simulink model "Controller_ABS_VLC_AYC"  (Simulink 8.7)
settings: Solver=ode3  SolverMode=SingleTasking  StartTime=0.0  StopTime=6  FixedStep=0.001  RelTol=1e-3
undefined symbols (not defined in the file): Lf, Lr, T_Avail
libraries: fuzblock x17, slrtlib x10, dspfdesign x5, simulink x4
settings Model: MinMaxOverflowLogging=ForceOff  Creator=MR Spyder  LastModifiedBy=kschmutz
settings DataIOCC: SignalLoggingSaveFormat=ModelDataLogs  SaveOutput=off  SaveTime=off
settings OptimizationCC: DefaultParameterBehavior=Inlined  ExpressionDepthLimit=2147483647
settings DebuggingCC: SolverPrmCheckMsg=warning  FcnCallInpInsideContextMsg=EnableAllAsWarning  StateNameClashWarn=warning
settings GRTTargetCC: CombineOutputUpdateFcns=off  GRTInterface=on

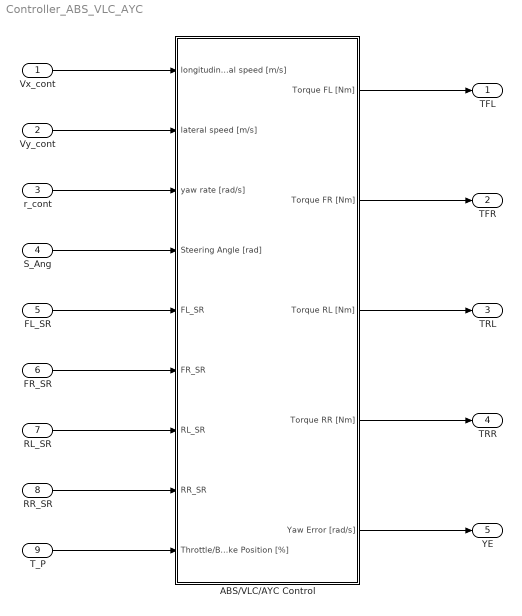
== system Controller_ABS_VLC_AYC ==
  Vx_cont : Inport
  Vy_cont : Inport  Port=2
  r_cont : Inport  Port=3
  S_Ang : Inport  Port=4
  FL_SR : Inport  Port=5
  FR_SR : Inport  Port=6
  RL_SR : Inport  Port=7
  RR_SR : Inport  Port=8
  T_P : Inport  Port=9
  ABS/VLC/AYC Control : Subsystem
  TFL : Outport
  TFR : Outport  Port=2
  TRL : Outport  Port=3
  TRR : Outport  Port=4
  YE : Outport  Port=5
  wires:
  T_P/1 -> ABS/VLC/AYC Control/9(Throttle/Brake Position [%])
  ABS/VLC/AYC Control/1(Torque FL [Nm]) -> TFL/1
  ABS/VLC/AYC Control/2(Torque FR [Nm]) -> TFR/1
  ABS/VLC/AYC Control/3(Torque RL [Nm]) -> TRL/1
  ABS/VLC/AYC Control/4(Torque RR [Nm]) -> TRR/1
  FL_SR/1 -> ABS/VLC/AYC Control/5(FL_SR)
  FR_SR/1 -> ABS/VLC/AYC Control/6(FR_SR)
  RL_SR/1 -> ABS/VLC/AYC Control/7(RL_SR)
  RR_SR/1 -> ABS/VLC/AYC Control/8(RR_SR)
  r_cont/1 -> ABS/VLC/AYC Control/3(yaw rate [rad/s])
  Vy_cont/1 -> ABS/VLC/AYC Control/2(lateral speed [m/s])
  Vx_cont/1 -> ABS/VLC/AYC Control/1(longitudinal speed [m/s])
  S_Ang/1 -> ABS/VLC/AYC Control/4(Steering Angle [rad])
  ABS/VLC/AYC Control/5(Yaw Error [rad/s]) -> YE/1

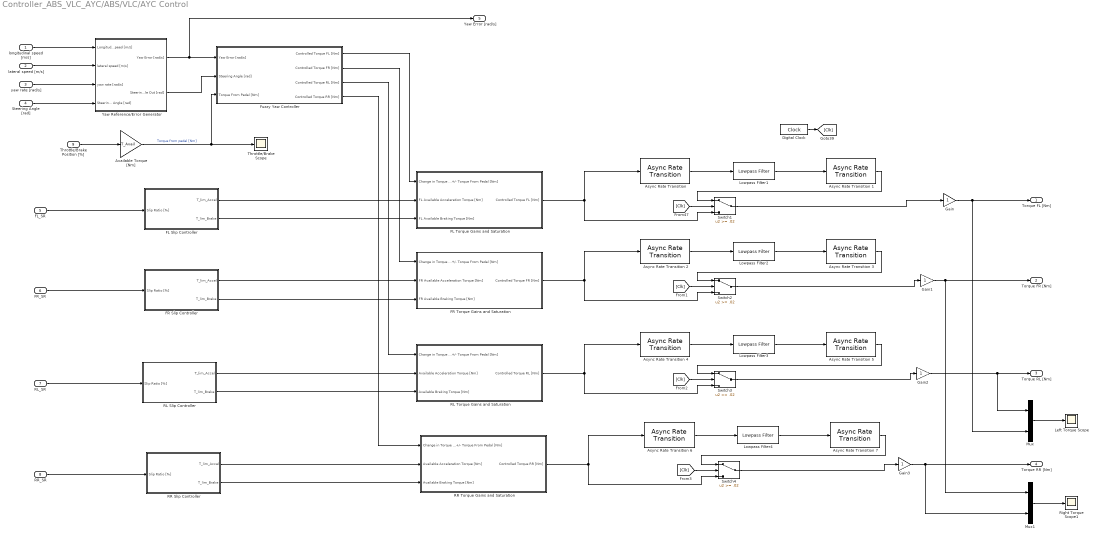
== system Controller_ABS_VLC_AYC/ABS/VLC/AYC Control ==
  longitudinal speed [m/s] : Inport
  lateral speed [m/s] : Inport  Port=2
  yaw rate [rad/s] : Inport  Port=3
  Steering Angle [rad] : Inport  Port=4
  FL_SR : Inport  Port=5
  FR_SR : Inport  Port=6
  RL_SR : Inport  Port=7
  RR_SR : Inport  Port=8
  Throttle/Brake Position [%] : Inport  Port=9
  Async Rate Transition {,1..7} (8 alike) : slrtlib/Asynchronous Event/Async Rate Transition   sample_time=0.001
  Available Torque [Nm] : Gain  Gain=T_Avail
  Digital Clock : DigitalClock  SampleTime=0.001
  FL Slip Controller : Subsystem
  FL Torque Gains and Saturation : Subsystem
  FR Slip Controller : Subsystem
  FR Torque Gains and Saturation : Subsystem
  Fuzzy Yaw Controller : Subsystem
  Gain{,1..3} (4 alike) : Gain
  Left Torque Scope : Scope
  Lowpass Filter{1..4} (4 alike) : dspfdesign/Lowpass Filter  FilterType=FIR  DesignForMinimumOrder=on  FilterOrder=50  PassbandFrequency=400  StopbandFrequency=499  PassbandRipple=0.1  StopbandAttenuation=80  InheritSampleRate=on  SampleRate=1000  roundingMode=Floor  coeffsDataTypeStr=fixdt(1,16)  SimulateUsing=Interpreted execution
  Mux : Mux  Inputs=2
  Mux1 : Mux  Inputs=2
  RL Slip Controller : Subsystem
  RL Torque Gains and Saturation : Subsystem
  RR Slip Controller : Subsystem
  RR Torque Gains and Saturation : Subsystem
  Right Torque Scope1 : Scope
  Switch{1..4} (4 alike) : Switch  Threshold=.02
  Throttle/Brake Scope : Scope
  Yaw Reference/Error Generator : Subsystem
  Torque FL [Nm] : Outport
  Torque FR [Nm] : Outport  Port=2
  Torque RL [Nm] : Outport  Port=3
  Torque RR [Nm] : Outport  Port=4
  Yaw Error [rad/s] : Outport  Port=5
  wires:
  Mux/1 -> Left Torque Scope/1
  longitudinal speed [m/s]/1 -> Yaw Reference/Error Generator/1(Longitudinal Speed [m/s])
  lateral speed [m/s]/1 -> Yaw Reference/Error Generator/2(lateral speed [m/s])
  yaw rate [rad/s]/1 -> Yaw Reference/Error Generator/3(yaw rate [rad/s])
  Steering Angle [rad]/1 -> Yaw Reference/Error Generator/4(Steering Angle [rad])
  Throttle/Brake Position [%]/1 -> Available Torque [Nm]/1
  Available Torque [Nm]/1 -> Fuzzy Yaw Controller/3(Torque From Pedal [Nm]), Throttle/Brake Scope/1  "Torque from pedal [Nm]"
  FL Slip Controller/2(T_lim_Brake) -> FL Torque Gains and Saturation/3(FL Available Braking Torque [Nm])
  Yaw Reference/Error Generator/1(Yaw Error [rad/s]) -> Yaw Error [rad/s]/1, Fuzzy Yaw Controller/1(Yaw Error [rad/s])
  Yaw Reference/Error Generator/2(Steering Angle Out [rad]) -> Fuzzy Yaw Controller/2(Steering Angle [rad])
  Fuzzy Yaw Controller/1(Controlled Torque FL [Nm]) -> FL Torque Gains and Saturation/1(Change in Torque +/- Torque From Pedal [Nm])
  Fuzzy Yaw Controller/2(Controlled Torque FR [Nm]) -> FR Torque Gains and Saturation/1(Change in Torque +/- Torque From Pedal [Nm])
  Fuzzy Yaw Controller/3(Controlled Torque RL [Nm]) -> RL Torque Gains and Saturation/1(Change in Torque +/- Torque From Pedal [Nm])
  Fuzzy Yaw Controller/4(Controlled Torque RR [Nm]) -> RR Torque Gains and Saturation/1(Change in Torque +/- Torque From Pedal [Nm])
  FR Slip Controller/1(T_lim_Accel) -> FR Torque Gains and Saturation/2(FR Available Acceleration Torque [Nm])
  FR Slip Controller/2(T_lim_Brake) -> FR Torque Gains and Saturation/3(FR Available Braking Torque [Nm])
  RL Slip Controller/1(T_lim_Accel) -> RL Torque Gains and Saturation/2(Available Acceleration Torque [Nm])
  RL Slip Controller/2(T_lim_Brake) -> RL Torque Gains and Saturation/3(Available Braking Torque [Nm])
  RR Slip Controller/1(T_lim_Accel) -> RR Torque Gains and Saturation/2(Available Acceleration Torque [Nm])
  RR Slip Controller/2(T_lim_Brake) -> RR Torque Gains and Saturation/3(Available Braking Torque [Nm])
  Mux1/1 -> Right Torque Scope1/1
  Gain/1 -> Torque FL [Nm]/1, Mux/2
  Gain1/1 -> Torque FR [Nm]/1, Mux1/1
  Gain2/1 -> Torque RL [Nm]/1, Mux/1
  Gain3/1 -> Torque RR [Nm]/1, Mux1/2
  FL_SR/1 -> FL Slip Controller/1(Slip Ratio [%])
  FR_SR/1 -> FR Slip Controller/1(Slip Ratio [%])
  RL_SR/1 -> RL Slip Controller/1(Slip Ratio [%])
  RR_SR/1 -> RR Slip Controller/1(Slip Ratio [%])
  FL Torque Gains and Saturation/1(Controlled Torque FL [Nm]) -> "Async Rate Transition "/1, Switch1/3
  FL Slip Controller/1(T_lim_Accel) -> FL Torque Gains and Saturation/2(FL Available Acceleration Torque [Nm])
  Lowpass Filter1/1 -> Async Rate Transition 1/1
  "Async Rate Transition "/1 -> Lowpass Filter1/1
  [Clk] -> Switch1/2
  Async Rate Transition 1/1 -> Switch1/1
  Switch1/1 -> Gain/1
  FR Torque Gains and Saturation/1(Controlled Torque FR [Nm]) -> Async Rate Transition 2/1, Switch2/3
  Lowpass Filter2/1 -> Async Rate Transition 3/1
  Async Rate Transition 2/1 -> Lowpass Filter2/1
  [Clk] -> Switch2/2
  Async Rate Transition 3/1 -> Switch2/1
  Switch2/1 -> Gain1/1
  RL Torque Gains and Saturation/1(Controlled Torque RL [Nm]) -> Async Rate Transition 4/1, Switch3/3
  Lowpass Filter3/1 -> Async Rate Transition 5/1
  Async Rate Transition 4/1 -> Lowpass Filter3/1
  [Clk] -> Switch3/2
  Async Rate Transition 5/1 -> Switch3/1
  Switch3/1 -> Gain2/1
  RR Torque Gains and Saturation/1(Controlled Torque RR [Nm]) -> Async Rate Transition 6/1, Switch4/3
  Lowpass Filter4/1 -> Async Rate Transition 7/1
  Async Rate Transition 6/1 -> Lowpass Filter4/1
  [Clk] -> Switch4/2
  Async Rate Transition 7/1 -> Switch4/1
  Switch4/1 -> Gain3/1
  Digital Clock/1 -> [Clk]

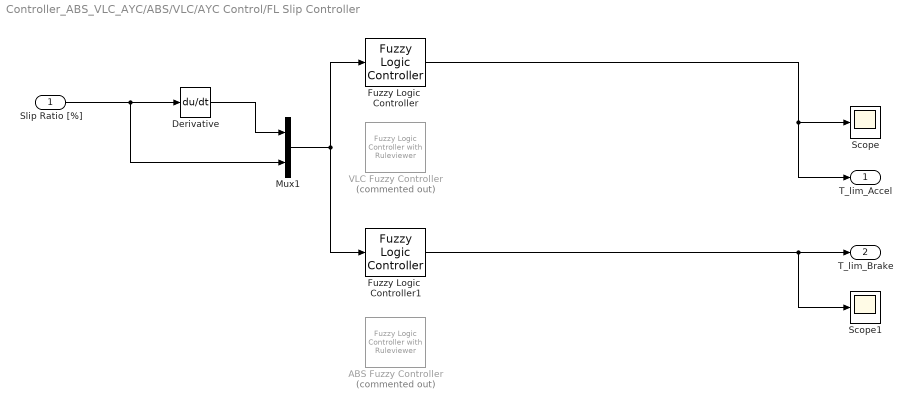
== system Controller_ABS_VLC_AYC/ABS/VLC/AYC Control/FL Slip Controller ==
  Slip Ratio [%] : Inport
  ABS Fuzzy Controller : fuzblock/Fuzzy Logic  Controller  with Ruleviewer  Commented=on  fismatrix=Fuzzy_Slip_Ctl_ABS  Ts=.1
  Derivative : Derivative
  Fuzzy Logic  Controller : fuzblock/Fuzzy Logic  Controller  fis=Fuzzy_Slip_Ctl_VLC
  Fuzzy Logic  Controller1 : fuzblock/Fuzzy Logic  Controller  fis=Fuzzy_Slip_Ctl_ABS
  Mux1 : Mux  Inputs=2
  Scope : Scope
  Scope1 : Scope
  VLC Fuzzy Controller : fuzblock/Fuzzy Logic  Controller  with Ruleviewer  Commented=on  fismatrix=Fuzzy_Slip_Ctl_VLC  Ts=.1
  T_lim_Accel : Outport
  T_lim_Brake : Outport  Port=2
  wires:
  Mux1/1 -> Fuzzy Logic  Controller/1, Fuzzy Logic  Controller1/1
  Slip Ratio [%]/1 -> Derivative/1, Mux1/2
  Derivative/1 -> Mux1/1
  Fuzzy Logic  Controller1/1 -> Scope1/1, T_lim_Brake/1
  Fuzzy Logic  Controller/1 -> T_lim_Accel/1, Scope/1

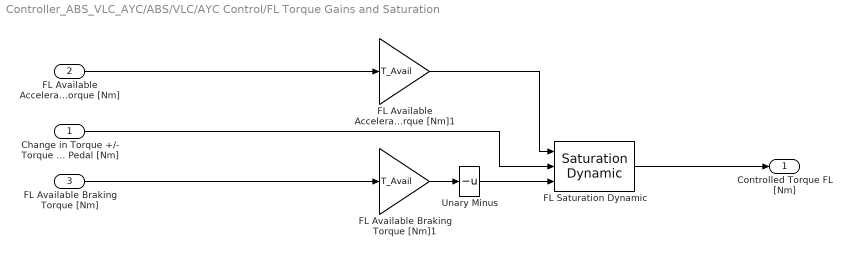
== system Controller_ABS_VLC_AYC/ABS/VLC/AYC Control/FL Torque Gains and Saturation ==
  Change in Torque +/- Torque From Pedal [Nm] : Inport
  FL Available Acceleration Torque [Nm] : Inport  Port=2
  FL Available Braking Torque [Nm] : Inport  Port=3
  FL Available Acceleration Torque [Nm]1 : Gain  Gain=T_Avail
  FL Available Braking Torque [Nm]1 : Gain  Gain=T_Avail
  FL Saturation Dynamic : simulink/Discontinuities/Saturation Dynamic  OutMin=[]  OutMax=[]  OutDataTypeStr=Inherit: Same as second input  OutDataType=fixdt(1, 16)  OutScaling=2^-10  DoSatur=off
  Unary Minus : UnaryMinus
  Controlled Torque FL [Nm] : Outport
  wires:
  FL Available Acceleration Torque [Nm]1/1 -> FL Saturation Dynamic/1
  Unary Minus/1 -> FL Saturation Dynamic/3
  FL Available Braking Torque [Nm]1/1 -> Unary Minus/1
  FL Available Acceleration Torque [Nm]/1 -> FL Available Acceleration Torque [Nm]1/1
  FL Available Braking Torque [Nm]/1 -> FL Available Braking Torque [Nm]1/1
  Change in Torque +/- Torque From Pedal [Nm]/1 -> FL Saturation Dynamic/2
  FL Saturation Dynamic/1 -> Controlled Torque FL [Nm]/1

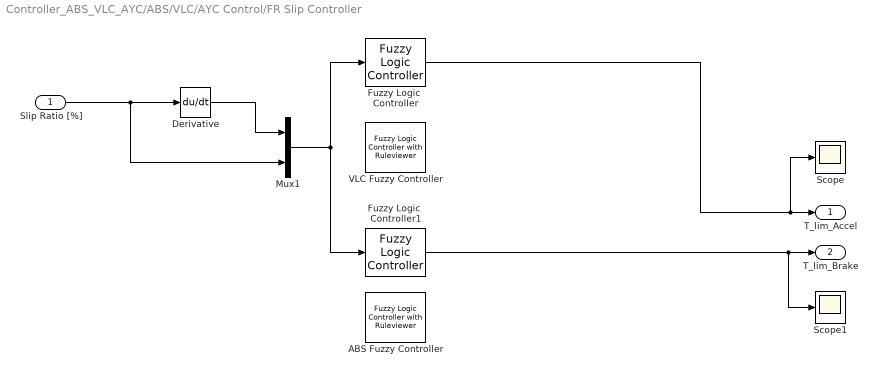
== system Controller_ABS_VLC_AYC/ABS/VLC/AYC Control/FR Slip Controller ==
  Slip Ratio [%] : Inport
  ABS Fuzzy Controller : fuzblock/Fuzzy Logic  Controller  with Ruleviewer  fismatrix=Fuzzy_Slip_Ctl_ABS  Ts=.1
  Derivative : Derivative
  Fuzzy Logic  Controller : fuzblock/Fuzzy Logic  Controller  fis=Fuzzy_Slip_Ctl_VLC
  Fuzzy Logic  Controller1 : fuzblock/Fuzzy Logic  Controller  fis=Fuzzy_Slip_Ctl_ABS
  Mux1 : Mux  Inputs=2
  Scope : Scope
  Scope1 : Scope
  VLC Fuzzy Controller : fuzblock/Fuzzy Logic  Controller  with Ruleviewer  fismatrix=Fuzzy_Slip_Ctl_VLC  Ts=.1
  T_lim_Accel : Outport
  T_lim_Brake : Outport  Port=2
  wires:
  Mux1/1 -> Fuzzy Logic  Controller/1, Fuzzy Logic  Controller1/1
  Slip Ratio [%]/1 -> Derivative/1, Mux1/2
  Derivative/1 -> Mux1/1
  Fuzzy Logic  Controller/1 -> Scope/1, T_lim_Accel/1
  Fuzzy Logic  Controller1/1 -> Scope1/1, T_lim_Brake/1

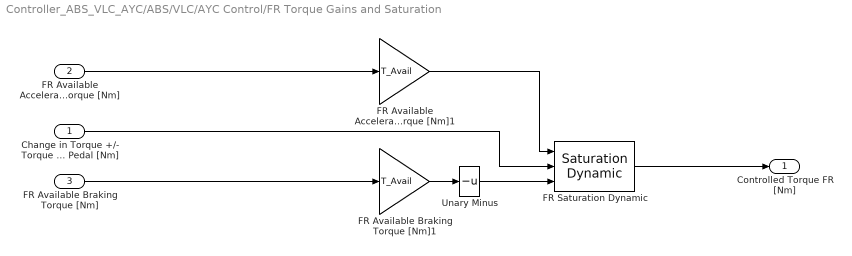
== system Controller_ABS_VLC_AYC/ABS/VLC/AYC Control/FR Torque Gains and Saturation ==
  Change in Torque +/- Torque From Pedal [Nm] : Inport
  FR Available Acceleration Torque [Nm] : Inport  Port=2
  FR Available Braking Torque [Nm] : Inport  Port=3
  FR Available Acceleration Torque [Nm]1 : Gain  Gain=T_Avail
  FR Available Braking Torque [Nm]1 : Gain  Gain=T_Avail
  FR Saturation Dynamic : simulink/Discontinuities/Saturation Dynamic  OutMin=[]  OutMax=[]  OutDataTypeStr=Inherit: Same as second input  OutDataType=fixdt(1, 16)  OutScaling=2^-10  DoSatur=off
  Unary Minus : UnaryMinus
  Controlled Torque FR [Nm] : Outport
  wires:
  FR Available Acceleration Torque [Nm]1/1 -> FR Saturation Dynamic/1
  Unary Minus/1 -> FR Saturation Dynamic/3
  FR Available Braking Torque [Nm]1/1 -> Unary Minus/1
  FR Available Acceleration Torque [Nm]/1 -> FR Available Acceleration Torque [Nm]1/1
  FR Available Braking Torque [Nm]/1 -> FR Available Braking Torque [Nm]1/1
  Change in Torque +/- Torque From Pedal [Nm]/1 -> FR Saturation Dynamic/2
  FR Saturation Dynamic/1 -> Controlled Torque FR [Nm]/1

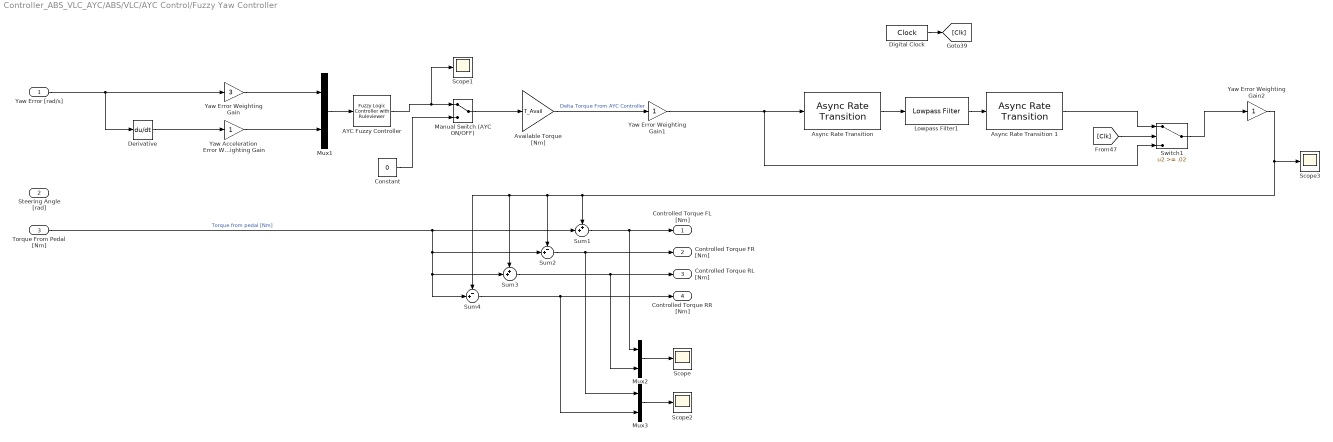
== system Controller_ABS_VLC_AYC/ABS/VLC/AYC Control/Fuzzy Yaw Controller ==
  Yaw Error [rad/s] : Inport
  Steering Angle [rad] : Inport  Port=2
  Torque From Pedal [Nm] : Inport  Port=3
  AYC Fuzzy Controller : fuzblock/Fuzzy Logic  Controller  with Ruleviewer  fismatrix=Fuzzy_AYC_Ctl  Ts=.1
  "Async Rate Transition " : slrtlib/Asynchronous Event/Async Rate Transition   sample_time=0.001
  Async Rate Transition 1 : slrtlib/Asynchronous Event/Async Rate Transition   sample_time=0.001
  Available Torque [Nm] : Gain  Gain=T_Avail
  Constant : Constant  Value=0
  Derivative : Derivative
  Digital Clock : DigitalClock  SampleTime=0.001
  Lowpass Filter1 : dspfdesign/Lowpass Filter  FilterType=FIR  DesignForMinimumOrder=on  FilterOrder=50  PassbandFrequency=400  StopbandFrequency=499  PassbandRipple=0.1  StopbandAttenuation=80  InheritSampleRate=on  SampleRate=1000  roundingMode=Floor  coeffsDataTypeStr=fixdt(1,16)  SimulateUsing=Interpreted execution
  Manual Switch (AYC ON/OFF) : ManualSwitch
  Mux1 : Mux  Inputs=2
  Mux2 : Mux  Inputs=2
  Mux3 : Mux  Inputs=2
  Scope{,1..3} (4 alike) : Scope
  Sum1 : Sum  Inputs=++|
  Sum2 : Sum  Inputs=-+|
  Sum3 : Sum  Inputs=++|
  Sum4 : Sum  Inputs=-+|
  Switch1 : Switch  Threshold=.02
  Yaw Acceleration Error Weighting Gain : Gain
  Yaw Error Weighting Gain : Gain  Gain=3
  Yaw Error Weighting Gain1 : Gain
  Yaw Error Weighting Gain2 : Gain
  Controlled Torque FL [Nm] : Outport
  Controlled Torque FR [Nm] : Outport  Port=2
  Controlled Torque RL [Nm] : Outport  Port=3
  Controlled Torque RR [Nm] : Outport  Port=4
  wires:
  Sum1/1 -> Controlled Torque FL [Nm]/1, Mux2/1
  Sum2/1 -> Controlled Torque FR [Nm]/1, Mux3/1
  Sum3/1 -> Controlled Torque RL [Nm]/1, Mux2/2
  Sum4/1 -> Controlled Torque RR [Nm]/1, Mux3/2
  Mux1/1 -> AYC Fuzzy Controller/1
  Yaw Error [rad/s]/1 -> Yaw Error Weighting Gain/1, Derivative/1
  Yaw Error Weighting Gain/1 -> Mux1/1
  Yaw Acceleration Error Weighting Gain/1 -> Mux1/2
  Mux2/1 -> Scope/1
  AYC Fuzzy Controller/1 -> Manual Switch (AYC ON/OFF)/1, Scope1/1
  Constant/1 -> Manual Switch (AYC ON/OFF)/2
  Manual Switch (AYC ON/OFF)/1 -> Available Torque [Nm]/1
  Mux3/1 -> Scope2/1
  Available Torque [Nm]/1 -> Yaw Error Weighting Gain1/1  "Delta Torque From AYC Controller"
  Derivative/1 -> Yaw Acceleration Error Weighting Gain/1
  Torque From Pedal [Nm]/1 -> Sum2/2, Sum3/2, Sum4/2, Sum1/2  "Torque from pedal [Nm]"
  Yaw Error Weighting Gain2/1 -> Scope3/1, Sum4/1, Sum3/1, Sum2/1, Sum1/1
  Yaw Error Weighting Gain1/1 -> Switch1/3, "Async Rate Transition "/1
  Lowpass Filter1/1 -> Async Rate Transition 1/1
  "Async Rate Transition "/1 -> Lowpass Filter1/1
  [Clk] -> Switch1/2
  Switch1/1 -> Yaw Error Weighting Gain2/1
  Async Rate Transition 1/1 -> Switch1/1
  Digital Clock/1 -> [Clk]

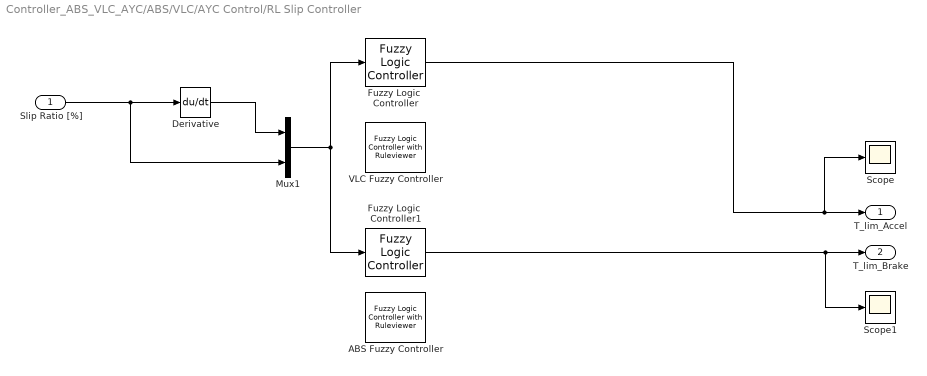
== system Controller_ABS_VLC_AYC/ABS/VLC/AYC Control/RL Slip Controller ==
  Slip Ratio [%] : Inport
  ABS Fuzzy Controller : fuzblock/Fuzzy Logic  Controller  with Ruleviewer  fismatrix=Fuzzy_Slip_Ctl_ABS  Ts=.1
  Derivative : Derivative
  Fuzzy Logic  Controller : fuzblock/Fuzzy Logic  Controller  fis=Fuzzy_Slip_Ctl_VLC
  Fuzzy Logic  Controller1 : fuzblock/Fuzzy Logic  Controller  fis=Fuzzy_Slip_Ctl_ABS
  Mux1 : Mux  Inputs=2
  Scope : Scope
  Scope1 : Scope
  VLC Fuzzy Controller : fuzblock/Fuzzy Logic  Controller  with Ruleviewer  fismatrix=Fuzzy_Slip_Ctl_VLC  Ts=.1
  T_lim_Accel : Outport
  T_lim_Brake : Outport  Port=2
  wires:
  Mux1/1 -> Fuzzy Logic  Controller/1, Fuzzy Logic  Controller1/1
  Slip Ratio [%]/1 -> Derivative/1, Mux1/2
  Derivative/1 -> Mux1/1
  Fuzzy Logic  Controller/1 -> Scope/1, T_lim_Accel/1
  Fuzzy Logic  Controller1/1 -> Scope1/1, T_lim_Brake/1

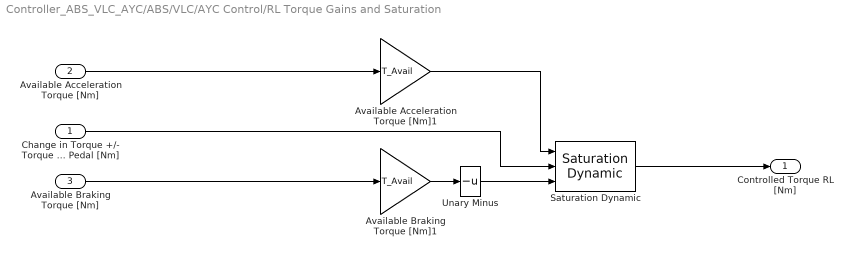
== system Controller_ABS_VLC_AYC/ABS/VLC/AYC Control/RL Torque Gains and Saturation ==
  Change in Torque +/- Torque From Pedal [Nm] : Inport
  Available Acceleration Torque [Nm] : Inport  Port=2
  Available Braking Torque [Nm] : Inport  Port=3
  Available Acceleration Torque [Nm]1 : Gain  Gain=T_Avail
  Available Braking Torque [Nm]1 : Gain  Gain=T_Avail
  Saturation Dynamic : simulink/Discontinuities/Saturation Dynamic  OutMin=[]  OutMax=[]  OutDataTypeStr=Inherit: Same as second input  OutDataType=fixdt(1, 16)  OutScaling=2^-10  DoSatur=off
  Unary Minus : UnaryMinus
  Controlled Torque RL [Nm] : Outport
  wires:
  Available Acceleration Torque [Nm]1/1 -> Saturation Dynamic/1
  Unary Minus/1 -> Saturation Dynamic/3
  Available Braking Torque [Nm]1/1 -> Unary Minus/1
  Available Acceleration Torque [Nm]/1 -> Available Acceleration Torque [Nm]1/1
  Available Braking Torque [Nm]/1 -> Available Braking Torque [Nm]1/1
  Change in Torque +/- Torque From Pedal [Nm]/1 -> Saturation Dynamic/2
  Saturation Dynamic/1 -> Controlled Torque RL [Nm]/1

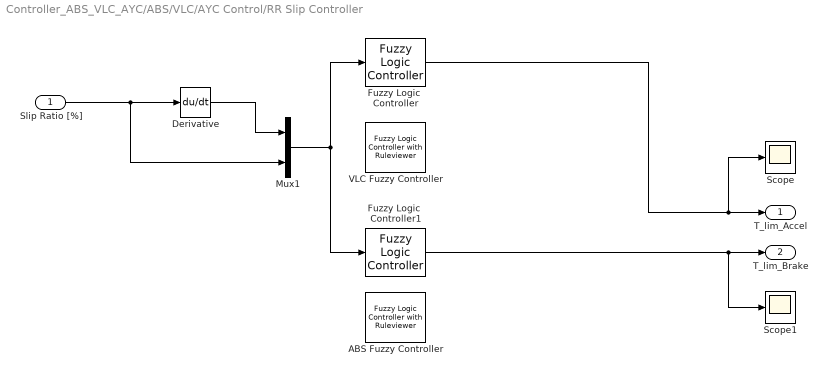
== system Controller_ABS_VLC_AYC/ABS/VLC/AYC Control/RR Slip Controller ==
  Slip Ratio [%] : Inport
  ABS Fuzzy Controller : fuzblock/Fuzzy Logic  Controller  with Ruleviewer  fismatrix=Fuzzy_Slip_Ctl_ABS  Ts=.1
  Derivative : Derivative
  Fuzzy Logic  Controller : fuzblock/Fuzzy Logic  Controller  fis=Fuzzy_Slip_Ctl_VLC
  Fuzzy Logic  Controller1 : fuzblock/Fuzzy Logic  Controller  fis=Fuzzy_Slip_Ctl_ABS
  Mux1 : Mux  Inputs=2
  Scope : Scope
  Scope1 : Scope
  VLC Fuzzy Controller : fuzblock/Fuzzy Logic  Controller  with Ruleviewer  fismatrix=Fuzzy_Slip_Ctl_VLC  Ts=.1
  T_lim_Accel : Outport
  T_lim_Brake : Outport  Port=2
  wires:
  Mux1/1 -> Fuzzy Logic  Controller/1, Fuzzy Logic  Controller1/1
  Slip Ratio [%]/1 -> Derivative/1, Mux1/2
  Derivative/1 -> Mux1/1
  Fuzzy Logic  Controller/1 -> Scope/1, T_lim_Accel/1
  Fuzzy Logic  Controller1/1 -> Scope1/1, T_lim_Brake/1

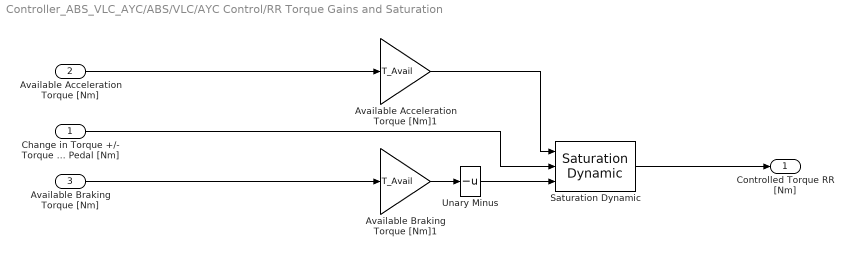
== system Controller_ABS_VLC_AYC/ABS/VLC/AYC Control/RR Torque Gains and Saturation ==
  Change in Torque +/- Torque From Pedal [Nm] : Inport
  Available Acceleration Torque [Nm] : Inport  Port=2
  Available Braking Torque [Nm] : Inport  Port=3
  Available Acceleration Torque [Nm]1 : Gain  Gain=T_Avail
  Available Braking Torque [Nm]1 : Gain  Gain=T_Avail
  Saturation Dynamic : simulink/Discontinuities/Saturation Dynamic  OutMin=[]  OutMax=[]  OutDataTypeStr=Inherit: Same as second input  OutDataType=fixdt(1, 16)  OutScaling=2^-10  DoSatur=off
  Unary Minus : UnaryMinus
  Controlled Torque RR [Nm] : Outport
  wires:
  Available Acceleration Torque [Nm]1/1 -> Saturation Dynamic/1
  Unary Minus/1 -> Saturation Dynamic/3
  Available Braking Torque [Nm]1/1 -> Unary Minus/1
  Available Acceleration Torque [Nm]/1 -> Available Acceleration Torque [Nm]1/1
  Available Braking Torque [Nm]/1 -> Available Braking Torque [Nm]1/1
  Change in Torque +/- Torque From Pedal [Nm]/1 -> Saturation Dynamic/2
  Saturation Dynamic/1 -> Controlled Torque RR [Nm]/1

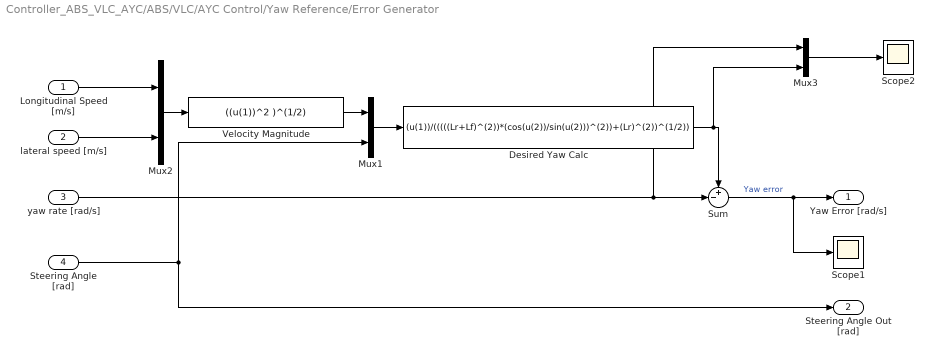
== system Controller_ABS_VLC_AYC/ABS/VLC/AYC Control/Yaw Reference/Error Generator ==
  Longitudinal Speed [m/s] : Inport
  lateral speed [m/s] : Inport  Port=2
  yaw rate [rad/s] : Inport  Port=3
  Steering Angle [rad] : Inport  Port=4
  Desired Yaw Calc : Fcn  Expr=(u(1))/(((((Lr+Lf)^(2))*(cos(u(2))/sin(u(2)))^(2))+(Lr)^(2))^(1/2))
  Mux1 : Mux  Inputs=2
  Mux2 : Mux  Inputs=2
  Mux3 : Mux  Inputs=2
  Scope1 : Scope
  Scope2 : Scope
  Sum : Sum  Inputs=+-|
  Velocity Magnitude : Fcn  Expr=((u(1))^2 )^(1/2)
  Yaw Error [rad/s] : Outport
  Steering Angle Out [rad] : Outport  Port=2
  wires:
  Mux1/1 -> Desired Yaw Calc/1
  lateral speed [m/s]/1 -> Mux2/2
  Longitudinal Speed [m/s]/1 -> Mux2/1
  Mux2/1 -> Velocity Magnitude/1
  Velocity Magnitude/1 -> Mux1/1
  Steering Angle [rad]/1 -> Mux1/2, Steering Angle Out [rad]/1
  yaw rate [rad/s]/1 -> Sum/2, Mux3/1
  Desired Yaw Calc/1 -> Sum/1, Mux3/2
  Sum/1 -> Yaw Error [rad/s]/1, Scope1/1  "Yaw error"
  Mux3/1 -> Scope2/1
